simulink model "iocmfac"  (R2021a)
settings: Solver=VariableStepAuto  StartTime=0.0  StopTime=250  RelTol=1e-3
settings Model: Creator=Lenovo  LastModifiedBy=Lenovo
settings SolverCC: AlgebraicLoopSolver=LineSearch
settings DataIOCC: ReturnWorkspaceOutputs=off
settings DebuggingCC: SFMachineParentedDataDiag=warning  ArithmeticOperatorsInVariantConditions=warning
settings SFSimCC: CustomCodeUndefinedFunction=UseInterfaceOnly

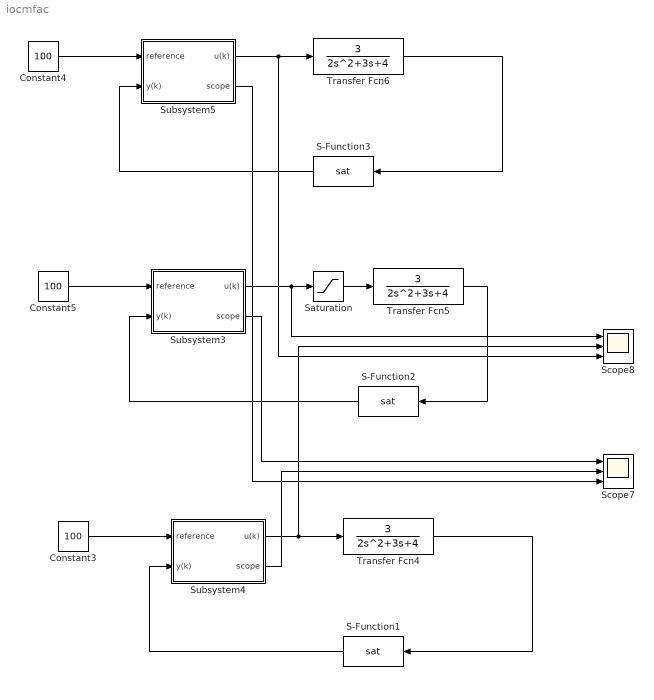
== system iocmfac ==
  Constant3 : Constant  Value=100
  Constant4 : Constant  Value=100
  Constant5 : Constant  Value=100
  S-Function1 : S-Function  FunctionName=sat  SFunctionDeploymentMode=off  EnableBusSupport=off
  S-Function2 : S-Function  FunctionName=sat  SFunctionDeploymentMode=off  EnableBusSupport=off
  S-Function3 : S-Function  FunctionName=sat  SFunctionDeploymentMode=off  EnableBusSupport=off
  Saturation : Saturate  UpperLimit=150
  Scope7 : Scope  NumInputPorts=3
  Scope8 : Scope  NumInputPorts=3
  Subsystem3 : Subsystem
  Subsystem4 : Subsystem
  Subsystem5 : Subsystem
  Transfer Fcn4 : TransferFcn  Numerator=[3]  Denominator=[2 3 4]
  Transfer Fcn5 : TransferFcn  Numerator=[3]  Denominator=[2 3 4]
  Transfer Fcn6 : TransferFcn  Numerator=[3]  Denominator=[2 3 4]
  wires:
  Subsystem3/1(u(k)) -> Scope8/1, Saturation/1
  Constant5/1 -> Subsystem3/1(reference)
  Transfer Fcn5/1 -> S-Function2/1
  S-Function2/1 -> Subsystem3/2(y(k))
  Constant3/1 -> Subsystem4/1(reference)
  Subsystem4/1(u(k)) -> Scope8/2, Transfer Fcn4/1
  S-Function1/1 -> Subsystem4/2(y(k))
  Transfer Fcn4/1 -> S-Function1/1
  Subsystem4/2(scope) -> Scope7/2
  Subsystem3/2(scope) -> Scope7/1
  S-Function3/1 -> Subsystem5/2(y(k))
  Constant4/1 -> Subsystem5/1(reference)
  Subsystem5/2(scope) -> Scope7/3
  Transfer Fcn6/1 -> S-Function3/1
  Subsystem5/1(u(k)) -> Scope8/3, Transfer Fcn6/1
  Saturation/1 -> Transfer Fcn5/1

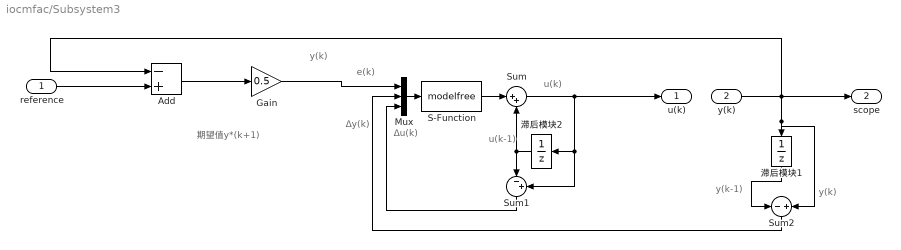
== system iocmfac/Subsystem3 ==
  note: y(k-1)
  note: y(k)
  note: e(k)
  note: Δu(k)
  note: u(k-1)
  note: u(k)
  note: Δy(k)
  note: y(k)
  note: 期望值y*(k+1)
  reference : Inport
  y(k) : Inport  Port=2
  Add : Sum  Inputs=-+
  Gain : Gain  Gain=0.5
  Mux : Mux  Inputs=3
  S-Function : S-Function  FunctionName=modelfree  Parameters=0.3,10,0.6  SFunctionDeploymentMode=off  EnableBusSupport=off
  Sum : Sum  Inputs=|++
  Sum1 : Sum  Inputs=|-+
  Sum2 : Sum  Inputs=-|+
  滞后模块1 : UnitDelay  SampleTime=-1  HasFrameUpgradeWarning=on
  滞后模块2 : UnitDelay  SampleTime=-1  HasFrameUpgradeWarning=on
  u(k) : Outport  VectorParamsAs1DForOutWhenUnconnected=off
  scope : Outport  Port=2  VectorParamsAs1DForOutWhenUnconnected=off
  wires:
  y(k)/1 -> scope/1, Sum2/2, 滞后模块1/1, Add/1
  滞后模块2/1 -> Sum1/1, Sum/2
  Sum2/1 -> Mux/2
  Mux/1 -> S-Function/1
  reference/1 -> Add/2
  S-Function/1 -> Sum/1
  滞后模块1/1 -> Sum2/1
  Sum1/1 -> Mux/3
  Add/1 -> Gain/1
  Sum/1 -> u(k)/1, 滞后模块2/1, Sum1/2
  Gain/1 -> Mux/1

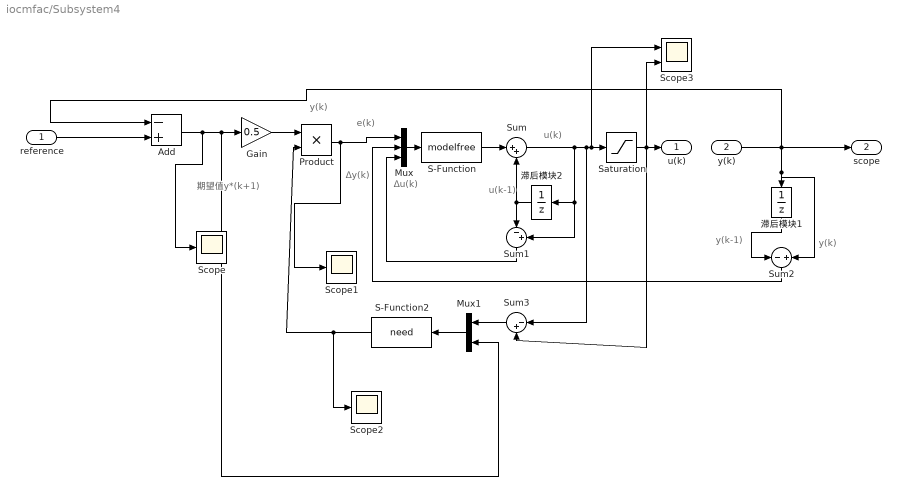
== system iocmfac/Subsystem4 ==
  note: y(k-1)
  note: y(k)
  note: e(k)
  note: Δu(k)
  note: u(k-1)
  note: u(k)
  note: Δy(k)
  note: y(k)
  note: 期望值y*(k+1)
  reference : Inport
  y(k) : Inport  Port=2
  Add : Sum  Inputs=-+
  Gain : Gain  Gain=0.5
  Mux : Mux  Inputs=3
  Mux1 : Mux  Inputs=2
  Product : Product
  S-Function : S-Function  FunctionName=modelfree  Parameters=0.3,10,0.6  SFunctionDeploymentMode=off  EnableBusSupport=off
  S-Function2 : S-Function  FunctionName=need  SFunctionDeploymentMode=off  EnableBusSupport=off
  Saturation : Saturate  UpperLimit=150
  Scope : Scope
  Scope1 : Scope
  Scope2 : Scope
  Scope3 : Scope  NumInputPorts=2
  Sum : Sum  Inputs=|++
  Sum1 : Sum  Inputs=|-+
  Sum2 : Sum  Inputs=-|+
  Sum3 : Sum  Inputs=|-+
  滞后模块1 : UnitDelay  SampleTime=-1  HasFrameUpgradeWarning=on
  滞后模块2 : UnitDelay  SampleTime=-1  HasFrameUpgradeWarning=on
  u(k) : Outport  VectorParamsAs1DForOutWhenUnconnected=off
  scope : Outport  Port=2  VectorParamsAs1DForOutWhenUnconnected=off
  wires:
  y(k)/1 -> scope/1, Sum2/2, 滞后模块1/1, Add/1
  滞后模块2/1 -> Sum1/1, Sum/2
  Sum/1 -> Sum3/1, Scope3/1, Saturation/1, 滞后模块2/1, Sum1/2
  Sum2/1 -> Mux/2
  Mux/1 -> S-Function/1
  reference/1 -> Add/2
  S-Function/1 -> Sum/1
  滞后模块1/1 -> Sum2/1
  Sum1/1 -> Mux/3
  Add/1 -> Scope/1, Mux1/2, Gain/1
  Saturation/1 -> Scope3/2, u(k)/1, Sum3/2
  Gain/1 -> Product/1
  Product/1 -> Scope1/1, Mux/1
  S-Function2/1 -> Scope2/1, Product/2
  Mux1/1 -> S-Function2/1
  Sum3/1 -> Mux1/1

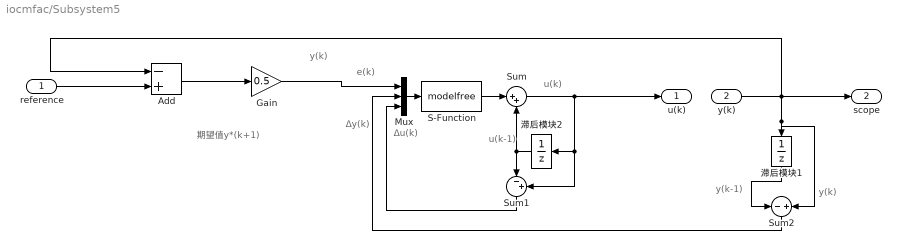
== system iocmfac/Subsystem5 ==
  note: y(k-1)
  note: y(k)
  note: e(k)
  note: Δu(k)
  note: u(k-1)
  note: u(k)
  note: Δy(k)
  note: y(k)
  note: 期望值y*(k+1)
  reference : Inport
  y(k) : Inport  Port=2
  Add : Sum  Inputs=-+
  Gain : Gain  Gain=0.5
  Mux : Mux  Inputs=3
  S-Function : S-Function  FunctionName=modelfree  Parameters=0.3,10,0.6  SFunctionDeploymentMode=off  EnableBusSupport=off
  Sum : Sum  Inputs=|++
  Sum1 : Sum  Inputs=|-+
  Sum2 : Sum  Inputs=-|+
  滞后模块1 : UnitDelay  SampleTime=-1  HasFrameUpgradeWarning=on
  滞后模块2 : UnitDelay  SampleTime=-1  HasFrameUpgradeWarning=on
  u(k) : Outport  VectorParamsAs1DForOutWhenUnconnected=off
  scope : Outport  Port=2  VectorParamsAs1DForOutWhenUnconnected=off
  wires:
  y(k)/1 -> scope/1, Sum2/2, 滞后模块1/1, Add/1
  滞后模块2/1 -> Sum1/1, Sum/2
  Sum2/1 -> Mux/2
  Mux/1 -> S-Function/1
  reference/1 -> Add/2
  S-Function/1 -> Sum/1
  滞后模块1/1 -> Sum2/1
  Sum1/1 -> Mux/3
  Add/1 -> Gain/1
  Sum/1 -> u(k)/1, 滞后模块2/1, Sum1/2
  Gain/1 -> Mux/1
